simulink model "que10_diode"  (R2020b)
settings: Solver=VariableStepAuto  StartTime=0.0  StopTime=1.99  RelTol=1e-3
model workspace (MAT data in the model file):
  V = [32.9 32.8 32.7 32.6 32.5 32.4 32.3 32.2 32.1 32 31.9 31.8 31.7 31.6 31.5 31.4 31.3 31.2 31.1 31 30.9 30.8 30.7 30.6 30.5 30.4 30.3 30.2 30.1 30 29.9 29.8 29.7 29.6 29.5 29.4 29.3 29.2 29.1 29 28.9 28.8 28.7 28.6 28.5 28.4 28.3 28.2 28.1 28 27.9 27.8 27.7 27.6 27.5 27.4 27.3 27.2 27.1 27 26.9 26.8 26.7 26.6 26.5 26.4 26.3 26.2 26.1 26 25.9 25.8 25.7 25.6 25.5 25.4 25.3 25.2 25.1 25 24.9 24.8 24.7 24.6 24.5 24.4 24.3 24.2 24.1 24 23.9 23.8 23.7 23.6 23.5 23.4 23.3 23.2 23.1 23 22.9 22.8 22.7 22.6 22.5 22.4 22.3 22.2 22.1 22 21.9 21.8 21.7 21.6 21.5 21.4 21.3 21.2 21.1 21 20.9 20.8 20.7 20.6 20.5 20.4 20.3 20.2 20.1 20 19.9 19.8 19.7 19.6 19.5 19.4 19.3 19.2 19.1 19 18.9 18.8 18.7 18.6 18.5 18.4 18.3 18.2 18.1 18 17.9 17.8 17.7 17.6 17.5 17.4 17.3 17.2 17.1 17 16.9 16.8 16.7 16.6 16.5 16.4 16.3 16.2 16.1 16 15.9 15.8 15.7 15.6 15.5 15.4 15.3 15.2 15.1 15 14.9 14.8 14.7 14.6 14.5 14.4 14.3 14.2 14.1 14 13.9 13.8 13.7 13.6 13.5 13.4 13.3 13.2 13.1 13 12.9 12.8 12.7 12.6 12.5 12.4 12.3 12.2 12.1 12 11.9 11.8 11.7 11.6 11.5 11.4 11.3 11.2 11.1 11 10.9 10.8 10.7 10.6 10.5 10.4 10.3 10.2 10.1 10 9.9 9.8 9.7 9.6 9.5 9.4 9.3 9.2 9.1 9 8.9 8.8 8.7 8.6 8.5 8.4 8.3 8.2 8.1 8 7.9 7.8 7.7 7.6 7.5 7.4 7.3 7.2 7.1 7 6.9 6.8 6.7 6.6 6.5 6.4 6.3 6.2 6.1 6 5.9 5.8 5.7 5.6 5.5 5.4 5.3 5.2 5.1 5 4.9 4.8 4.7 4.6 4.5 4.4 4.3 4.2 4.1 4 3.9 3.8 3.7 3.6 3.5 3.4 3.3 3.2 3.1 3 2.9 2.8 2.7 2.6 2.5 2.4 2.3 2.2 2.1 2 1.9 1.8 1.7 1.6 1.5 1.4 1.3 1.2 1.1 1 0.9 0.8 0.7 0.6 0.5 0.4 0.3 0.2 0.1 0]
libraries: simulink x3
settings Model: Creator=hp  LastModifiedBy=hp

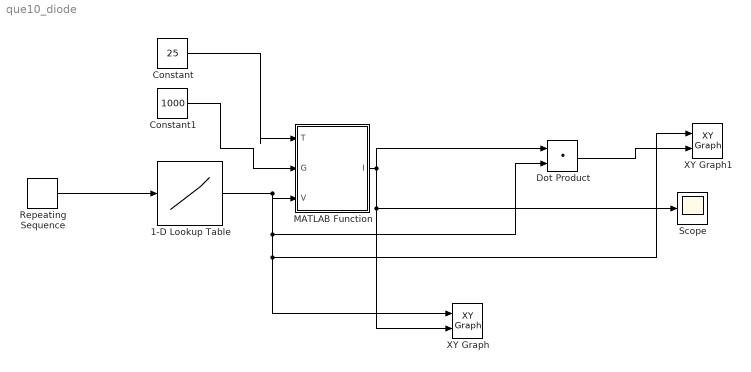
== system que10_diode ==
  1-D Lookup Table : Lookup_n-D  NumberOfTableDimensions=1  BreakpointsForDimension1=[1:330]  Table=V([1:330])  InternalRulePriority=Speed  RndMeth=Simplest
  Constant : Constant  Value=25
  Constant1 : Constant  Value=1000
  Dot Product : DotProduct  InputSameDT=on  OutDataTypeStr=Inherit: Inherit via internal rule
  MATLAB Function : MATLAB Function  TreatAsAtomicUnit=on
  Repeating Sequence : simulink/Sources/Repeating Sequence  rep_seq_t=[0 2]  rep_seq_y=[0 2]
  Scope : Scope
  XY Graph : simulink/Sinks/XY Graph  xmin=0  xmax=40  ymin=0  ymax=10  st=-1
  XY Graph1 : simulink/Sinks/XY Graph  xmin=-1  xmax=1  ymin=-1  ymax=1  st=-1
  wires:
  Constant/1 -> MATLAB Function/1(T)
  Constant1/1 -> MATLAB Function/2(G)
  Repeating Sequence/1 -> 1-D Lookup Table/1
  1-D Lookup Table/1 -> XY Graph/1, XY Graph1/1, Dot Product/2, MATLAB Function/3(V)
  MATLAB Function/1(I) -> Scope/1, XY Graph/2, Dot Product/1
  Dot Product/1 -> XY Graph1/2

== matlab function que10_diode/MATLAB Function ==
  data: T input; I output; G input; V input
function I = fcn(T,G,V)

K=1.38065e-23; %boltzman constant
q=1.602e-19; %charge of electron
Iscn=8.21;
Vocn=32.9;
%Kv=-0.123;
Ki=0.0032;
Ns=54;
T=T+273;
Tn=25+273;
Gn=1050;
a=1.3;
Eg=1.12;
%G=1000;
Rs=0.221;
Rp=415.405;


I=0;

Vtn=Ns*(K*Tn/q);
Ion= Iscn/((exp(Vocn/(a*Vtn)))-1);
Io_part=((q*Eg/(a*K))*((1/Tn)-(1/T)));
Io=Ion*((Tn/T)^3)*exp(Io_part);

Ipvn=Iscn;
Ipv=(Ipvn+Ki*(T-Tn))*(G/Gn);
Vt=Ns*(K*T/q);
I_part=Io*(exp((V+(I*Rs))/(Vt*a))-1)+((V+(Rs*I))/Rp);
I=Ipv-I_part;
